simulink model "Avionics"  (R2023b)
settings: Solver=FixedStepAuto  StartTime=0.0  StopTime=75  FixedStep=0.016666666666666666  RelTol=1e-3  EnableMultiTasking=on
PreLoadFcn:
  | load asbSkyHoggData.mat
model workspace (MAT data in the model file):
  Tc = 0.0166666666667
  Ts = 0
  cg_0 = [2.158 0 0]
  g_0 = [0 0 9.81]
libraries: aerolibnav x1
settings Model: DataDictionary=interfaces.sldd  Creator=The MathWorks, Inc.  LastModifiedBy=Gamax
settings SolverCC: AlgebraicLoopSolver=TrustRegion  MaxZcPerStep=1
settings DataIOCC: ExternalInput=getinputstruct(op_skyhogg3dof2V5)  InitialState=getstatestruct(op_skyhogg3dof2V5)  LimitDataPoints=on  SaveFormat=StructureWithTime  SaveOutput=off  SaveTime=off  ReturnWorkspaceOutputs=off
settings OptimizationCC: BlockReduction=off  BufferReuse=off  ExpressionDepthLimit=2147483647  InitFltsAndDblsToZero=on  LifeSpan=inf
settings DebuggingCC: WriteAfterWriteMsg=DisableAll  AlgebraicLoopMsg=none  SaveWithParameterizedLinksMsg=none  SignalResolutionControl=TryResolveAllWithWarning  FcnCallInpInsideContextMsg=warning  UniqueDataStoreMsg=error  AllowSymbolicDim=off  StateNameClashWarn=warning  SubsystemReferenceDiagnosticForUnitTest=warning  StrictBusMsg=ErrorOnBusTreatedAsVector  SFUnexpectedBacktrackingDiag=warning  SFNoUnconditionalDefaultTransitionDiag=warning  SFExecutionAtInitializationDiag=none  ArithmeticOperatorsInVariantConditions=warning
settings HardwareCC: ProdBitPerPointer=32  ProdBitPerSizeT=32  ProdBitPerPtrDiffT=32  ProdLargestAtomicFloat=None  ProdIntDivRoundTo=Undefined  ProdEndianess=Unspecified  ProdWordSize=32  ProdHWDeviceType=32-bit Generic
settings ModelReferenceCC: EnableRefExpFcnMdlSchedulingChecks=on  PropagateSignalLabelsOutOfModel=off
settings SFSimCC: SimUseLocalCustomCode=off  CustomCodeUndefinedFunction=UseInterfaceOnly
settings RTWCC: RTWUseLocalCustomCode=off  DLArmComputeVersion=19.05
settings CodeAppCC: StateflowObjectComments=on
settings GRTTargetCC: TargetFcnLib=ansi_tfl_tmw.mat  TargetLangStandard=C89/C90 (ANSI)  CombineOutputUpdateFcns=off  GRTInterface=on
settings ConfigComp: CovMetricSettings=dw  CovSaveCumulativeToWorkspaceVar=on  CovSaveSingleToWorkspaceVar=on  CovExternalEMLEnable=off  CovSFcnEnable=off

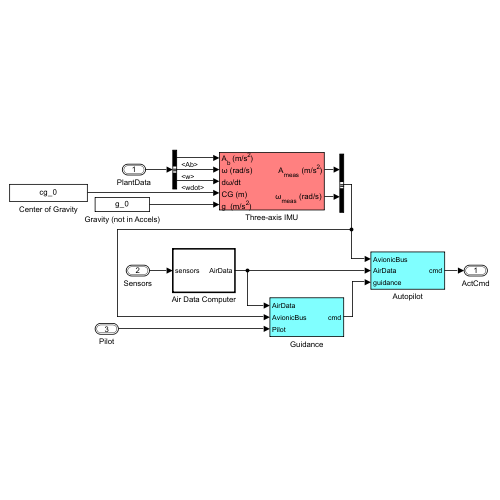
[thumbnail: Simulink's stored preview of the top-level diagram]
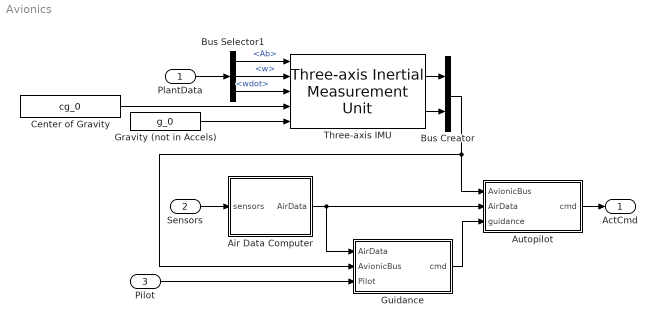
== system Avionics ==
  PlantData : Inport  OutDataTypeStr=Bus: PlantDataBus  SampleTime=Tc
  Sensors : Inport  Port=2  OutDataTypeStr=Bus: SensorDataBus  SampleTime=Tc
  Pilot : Inport  Port=3  OutDataTypeStr=Bus: PilotCmdBus  SampleTime=Tc
  Air Data Computer : Subsystem  TreatAsAtomicUnit=on
  Autopilot : Subsystem
  Bus Creator : BusCreator  Inputs=2
  Bus Selector1 : BusSelector  OutputSignals=Ab,w,wdot
  Center of Gravity : Constant  Value=cg_0  SampleTime=Tc
  Gravity (not in Accels) : Constant  Value=g_0  SampleTime=Tc
  Guidance : Subsystem
  Three-axis IMU : aerolibnav/Three-axis Inertial Measurement Unit  units=Metric (MKS)  imu=cg_0  i_Ts=Tc  dtype_a=off  w_a=190  z_a=0.707  a_sf_cc=[1 0 0; 0 1 0; 0 0 1]  a_bias=[0 0 0]  a_sat="[-inf  -inf  -inf  inf inf inf]"  dtype_g=off  w_g=190  z_g=0.707  g_sf_cc=[1 0 0; 0 1 0; 0 0 1]  g_bias=[0 0 0]  g_sens=[0 0 0]  g_sat="[-inf  -inf  -inf  inf inf inf]"  i_rand=off  i_seeds=[23093 23094 23095 23096 23097 23098]  i_pow=[0.001 0.001 0.001 0.0001 0.0001 0.0001]
  ActCmd : Outport  OutDataTypeStr=Bus: ActuatorCmdBus  SampleTime=Tc  VectorParamsAs1DForOutWhenUnconnected=off
  wires:
  Autopilot/1(cmd) -> ActCmd/1
  Three-axis IMU/2 -> Bus Creator/2
  Three-axis IMU/1 -> Bus Creator/1
  Bus Selector1/1 -> Three-axis IMU/1  "<Ab>"
  Center of Gravity/1 -> Three-axis IMU/4
  Bus Selector1/2 -> Three-axis IMU/2  "<w>"
  Bus Creator/1 -> Guidance/2(AvionicBus), Autopilot/1(AvionicBus)
  Gravity (not in Accels)/1 -> Three-axis IMU/5
  Guidance/1(cmd) -> Autopilot/3(guidance)
  Air Data Computer/1(AirData) -> Guidance/1(AirData), Autopilot/2(AirData)
  PlantData/1 -> Bus Selector1/1
  Pilot/1 -> Guidance/3(Pilot)
  Bus Selector1/3 -> Three-axis IMU/3  "<wdot>"
  Sensors/1 -> Air Data Computer/1(sensors)

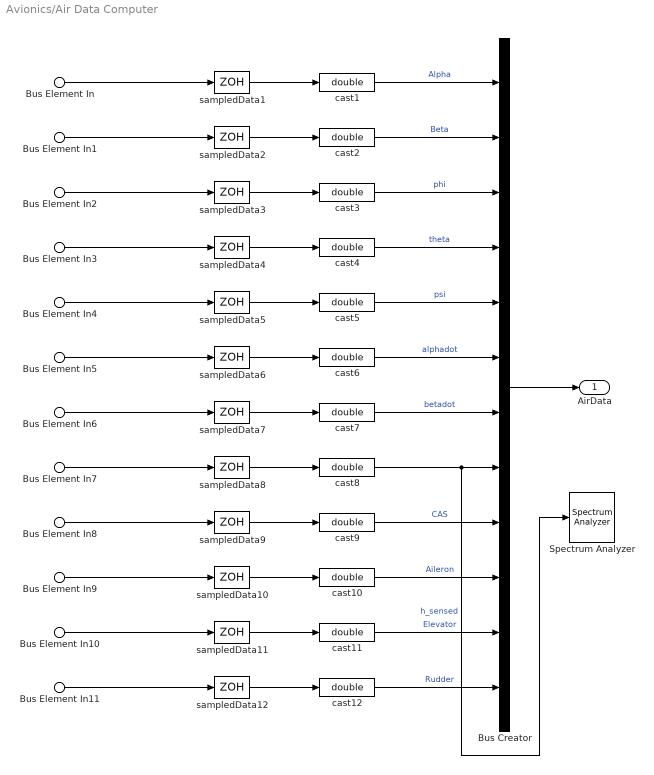
== system Avionics/Air Data Computer ==
  Bus Element In9 : Inport  PortName=sensors  Element=ActPositions.Aileron
  Bus Element In10 : Inport  PortName=sensors  Element=ActPositions.Elevator
  Bus Element In11 : Inport  PortName=sensors  Element=ActPositions.Rudder
  Bus Element In2 : Inport  PortName=sensors  Element=bodyAngles.phi
  Bus Element In3 : Inport  PortName=sensors  Element=bodyAngles.theta
  Bus Element In4 : Inport  PortName=sensors  Element=bodyAngles.psi
  Bus Element In : Inport  PortName=sensors  Element=alpha
  Bus Element In1 : Inport  PortName=sensors  Element=beta
  Bus Element In5 : Inport  PortName=sensors  Element=alphadot
  Bus Element In6 : Inport  PortName=sensors  Element=betadot
  Bus Element In7 : Inport  PortName=sensors  Element=h_sensed
  Bus Element In8 : Inport  PortName=sensors  Element=airSpeedCalibrated
  Bus Creator : BusCreator  Inputs=12
  Spectrum Analyzer : SpectrumAnalyzer  WindowPosition=[880.000000,470.000000,800.000000,500.000000,]  Visible=on  ScopeFrameLocation=window  SampleRateSource=Property  SampleRate=60  PlotAsTwoSidedSpectrum=off  FrequencyScale=Log  StartFrequency=20  StopFrequency=20e3  YLimits=[-133.32224754,11.62068091]
  cast{1..12} (12 alike) : DataTypeConversion  OutDataTypeStr=double  SaturateOnIntegerOverflow=off  RndMeth=Floor
  sampledData{1..12} (12 alike) : ZeroOrderHold  SampleTime=Tc
  AirData : Outport  VectorParamsAs1DForOutWhenUnconnected=off
  wires:
  cast11/1 -> Bus Creator/11  "Elevator"
  Bus Element In10/1 -> sampledData11/1
  sampledData12/1 -> cast12/1
  sampledData11/1 -> cast11/1
  Bus Element In11/1 -> sampledData12/1
  Bus Element In9/1 -> sampledData10/1
  Bus Element In8/1 -> sampledData9/1
  Bus Element In7/1 -> sampledData8/1
  Bus Element In6/1 -> sampledData7/1
  Bus Element In5/1 -> sampledData6/1
  Bus Element In4/1 -> sampledData5/1
  Bus Element In3/1 -> sampledData4/1
  Bus Element In2/1 -> sampledData3/1
  Bus Element In1/1 -> sampledData2/1
  Bus Element In/1 -> sampledData1/1
  cast4/1 -> Bus Creator/4  "theta"
  sampledData10/1 -> cast10/1
  sampledData9/1 -> cast9/1
  sampledData8/1 -> cast8/1
  sampledData7/1 -> cast7/1
  sampledData6/1 -> cast6/1
  sampledData5/1 -> cast5/1
  sampledData4/1 -> cast4/1
  sampledData3/1 -> cast3/1
  sampledData2/1 -> cast2/1
  sampledData1/1 -> cast1/1
  cast5/1 -> Bus Creator/5  "psi"
  cast6/1 -> Bus Creator/6  "alphadot"
  cast7/1 -> Bus Creator/7  "betadot"
  cast8/1 -> Spectrum Analyzer/1, Bus Creator/8  "h_sensed"
  cast9/1 -> Bus Creator/9  "CAS"
  cast10/1 -> Bus Creator/10  "Aileron"
  cast12/1 -> Bus Creator/12  "Rudder"
  cast3/1 -> Bus Creator/3  "phi"
  cast2/1 -> Bus Creator/2  "Beta"
  cast1/1 -> Bus Creator/1  "Alpha"
  Bus Creator/1 -> AirData/1

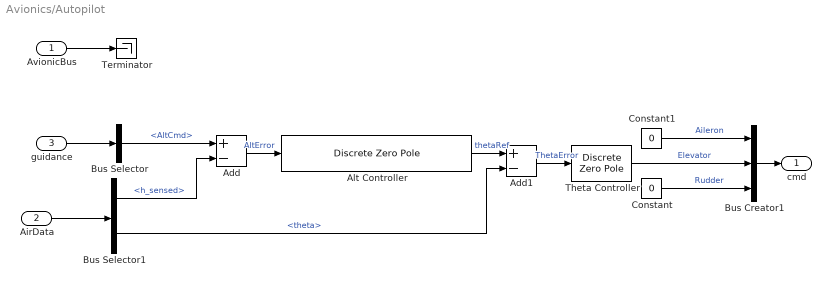
== system Avionics/Autopilot ==
  AvionicBus : Inport
  AirData : Inport  Port=2
  guidance : Inport  Port=3
  Add : Sum  Inputs=+-
  Add1 : Sum  Inputs=+-
  Alt Controller : DiscreteZeroPole  Zeros=[0.998853192323097;0.977076159863424]  Poles=[1;0.980841826994512]  Gain=0.0337283240400683*0.1  SampleTime=Tc
  Bus Creator1 : BusCreator  Inputs=3  OutDataTypeStr=Bus: ActuatorCmdBus
      settings: InheritFromInputs=off
  Bus Selector : BusSelector  OutputSignals=AltCmd
  Bus Selector1 : BusSelector  OutputSignals=h_sensed,theta
  Constant : Constant  Value=0  SampleTime=Tc
  Constant1 : Constant  Value=0  SampleTime=Tc
  Terminator : Terminator
  Theta Controller : DiscreteZeroPole  Zeros=0.999268009521977  Poles=1  Gain=-261.8699347622  SampleTime=Tc
  cmd : Outport  SampleTime=Tc  VectorParamsAs1DForOutWhenUnconnected=off
  wires:
  Bus Selector1/2 -> Add1/2  "<theta>"
  Bus Selector1/1 -> Add/2  "<h_sensed>"
  Constant1/1 -> Bus Creator1/1  "Aileron"
  Theta Controller/1 -> Bus Creator1/2  "Elevator"
  Constant/1 -> Bus Creator1/3  "Rudder"
  Bus Creator1/1 -> cmd/1
  AvionicBus/1 -> Terminator/1
  AirData/1 -> Bus Selector1/1
  guidance/1 -> Bus Selector/1
  Bus Selector/1 -> Add/1  "<AltCmd>"
  Add/1 -> Alt Controller/1  "AltError"
  Alt Controller/1 -> Add1/1  "thetaRef"
  Add1/1 -> Theta Controller/1  "ThetaError"

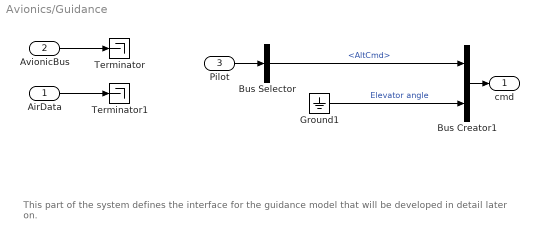
== system Avionics/Guidance ==
  note: This part of the system defines the interface for the guidance model that will be developed in detail later on.
  AirData : Inport
  AvionicBus : Inport  Port=2
  Pilot : Inport  Port=3
  Bus Creator1 : BusCreator  Inputs=2
  Bus Selector : BusSelector  OutputSignals=AltCmd
  Ground1 : Ground
  Terminator : Terminator
  Terminator1 : Terminator
  cmd : Outport  VectorParamsAs1DForOutWhenUnconnected=off
  wires:
  AirData/1 -> Terminator1/1
  AvionicBus/1 -> Terminator/1
  Bus Creator1/1 -> cmd/1
  Ground1/1 -> Bus Creator1/2  "Elevator angle"
  Bus Selector/1 -> Bus Creator1/1  "<AltCmd>"
  Pilot/1 -> Bus Selector/1
